simulink model "model_knigge"  (R2020b)
settings: configuration reference "Configuration" (kept outside this file)
settings Model: Creator=dogukan  LastModifiedBy=dogukan
settings ConfigSetRef: SourceName=Configuration  SourceLocation=Base Workspace

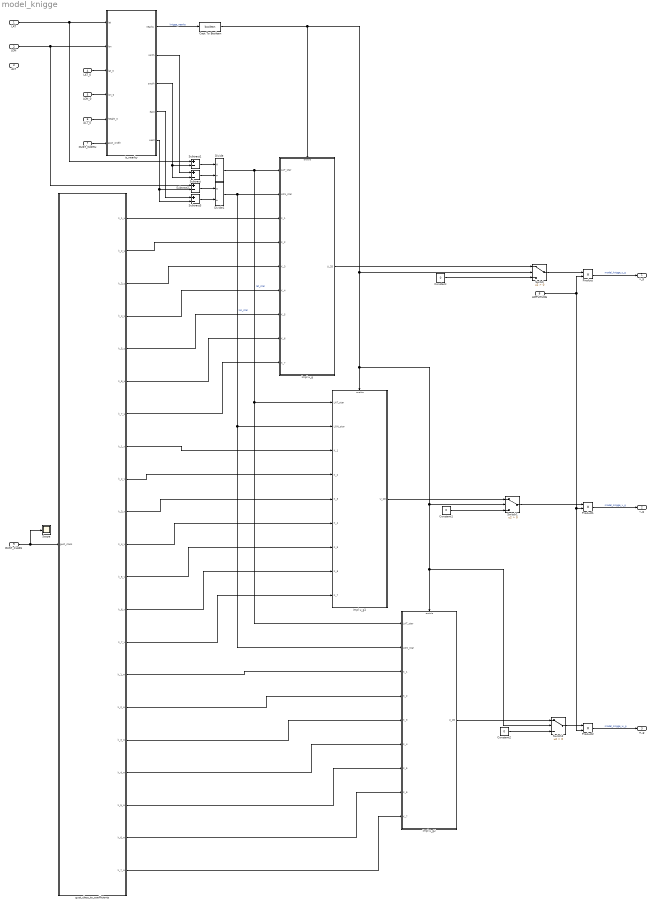
== system model_knigge ==
  LAT : Inport
  LON : Inport  Port=2
  ALT : Inport  Port=3
  LAT_0 : Inport  Port=4
  LON_0 : Inport  Port=5
  ALT_0 : Inport  Port=6
  GUST_WIDTH : Inport  Port=7
  AMPLITUDE : Inport  Port=8
  GUST_CLASS : Inport  Port=9
  Cast To Boolean : DataTypeConversion  OutDataTypeStr=boolean
  Constant : Constant  Value=0
  Constant1 : Constant  Value=0
  Constant2 : Constant  Value=0
  Divide : Product  Inputs=*/
  Divide1 : Product  Inputs=*/
  Product : Product
  Product1 : Product
  Product2 : Product
  Scope : Scope
  Subtract{,1..3} (4 alike) : Sum  Inputs=+-
  Switch : Switch  Criteria=u2 > Threshold
  Switch1 : Switch  Criteria=u2 > Threshold
  Switch2 : Switch  Criteria=u2 > Threshold
  gust_class_to_coefficients : MATLAB Function  TreatAsAtomicUnit=on
  impl u_g : Subsystem  TreatAsAtomicUnit=on
  impl u_g1 : Subsystem  TreatAsAtomicUnit=on
  impl u_g2 : Subsystem  TreatAsAtomicUnit=on
  is_nearby : MATLAB Function  TreatAsAtomicUnit=on
  u_g : Outport
  v_g : Outport  Port=2
  w_g : Outport  Port=3
  wires:
  LAT/1 -> is_nearby/1(lat), Subtract1/1
  LON/1 -> is_nearby/2(lon), Subtract2/1
  is_nearby/1(nearby) -> Cast To Boolean/1  "knigge_nearby"
  impl u_g/1(U_2D) -> Switch/1
  Cast To Boolean/1 -> impl u_g/Enable, impl u_g2/Enable, Switch2/2, Switch1/2, impl u_g1/Enable, Switch/2
  Constant/1 -> Switch/3
  LAT_0/1 -> is_nearby/3(lat_0)
  LON_0/1 -> is_nearby/4(lon_0)
  ALT_0/1 -> is_nearby/5(height_0)
  GUST_WIDTH/1 -> is_nearby/6(gust_width)
  Divide/1 -> impl u_g2/1(LAT_star), impl u_g1/1(LAT_star), impl u_g/1(LAT_star)  "lat_star"
  is_nearby/2(north) -> Subtract/1
  is_nearby/3(south) -> Subtract/2, Subtract1/2
  Subtract/1 -> Divide/2
  Subtract1/1 -> Divide/1
  Divide1/1 -> impl u_g2/2(LON_star), impl u_g1/2(LON_star), impl u_g/2(LON_star)  "lon_star"
  Subtract2/1 -> Divide1/1
  Subtract3/1 -> Divide1/2
  is_nearby/4(east) -> Subtract3/1
  is_nearby/5(west) -> Subtract3/2, Subtract2/2
  gust_class_to_coefficients/2(k_2_u) -> impl u_g/4(K_2)
  gust_class_to_coefficients/1(k_1_u) -> impl u_g/3(K_1)
  gust_class_to_coefficients/3(k_3_u) -> impl u_g/5(K_3)
  gust_class_to_coefficients/4(k_4_u) -> impl u_g/6(K_4)
  gust_class_to_coefficients/5(k_5_u) -> impl u_g/7(K_5)
  gust_class_to_coefficients/6(k_6_u) -> impl u_g/8(K_6)
  gust_class_to_coefficients/7(k_7_u) -> impl u_g/9(K_7)
  GUST_CLASS/1 -> Scope/1, gust_class_to_coefficients/1(gust_class)
  gust_class_to_coefficients/8(k_1_v) -> impl u_g1/3(K_1)
  gust_class_to_coefficients/9(k_2_v) -> impl u_g1/4(K_2)
  gust_class_to_coefficients/10(k_3_v) -> impl u_g1/5(K_3)
  gust_class_to_coefficients/11(k_4_v) -> impl u_g1/6(K_4)
  gust_class_to_coefficients/12(k_5_v) -> impl u_g1/7(K_5)
  gust_class_to_coefficients/13(k_6_v) -> impl u_g1/8(K_6)
  gust_class_to_coefficients/14(k_7_v) -> impl u_g1/9(K_7)
  impl u_g1/1(U_2D) -> Switch1/1
  Constant1/1 -> Switch1/3
  Switch1/1 -> Product1/1
  gust_class_to_coefficients/15(k_1_w) -> impl u_g2/3(K_1)
  gust_class_to_coefficients/16(k_2_w) -> impl u_g2/4(K_2)
  gust_class_to_coefficients/17(k_3_w) -> impl u_g2/5(K_3)
  gust_class_to_coefficients/18(k_4_w) -> impl u_g2/6(K_4)
  gust_class_to_coefficients/19(k_5_w) -> impl u_g2/7(K_5)
  gust_class_to_coefficients/20(k_6_w) -> impl u_g2/8(K_6)
  gust_class_to_coefficients/21(k_7_w) -> impl u_g2/9(K_7)
  impl u_g2/1(U_2D) -> Switch2/1
  Constant2/1 -> Switch2/3
  Switch2/1 -> Product2/1
  Switch/1 -> Product/1
  Product/1 -> u_g/1  "model_knigge_u_g"
  AMPLITUDE/1 -> Product2/2, Product1/2, Product/2
  Product1/1 -> v_g/1  "model_knigge_v_g"
  Product2/1 -> w_g/1  "model_knigge_w_g"

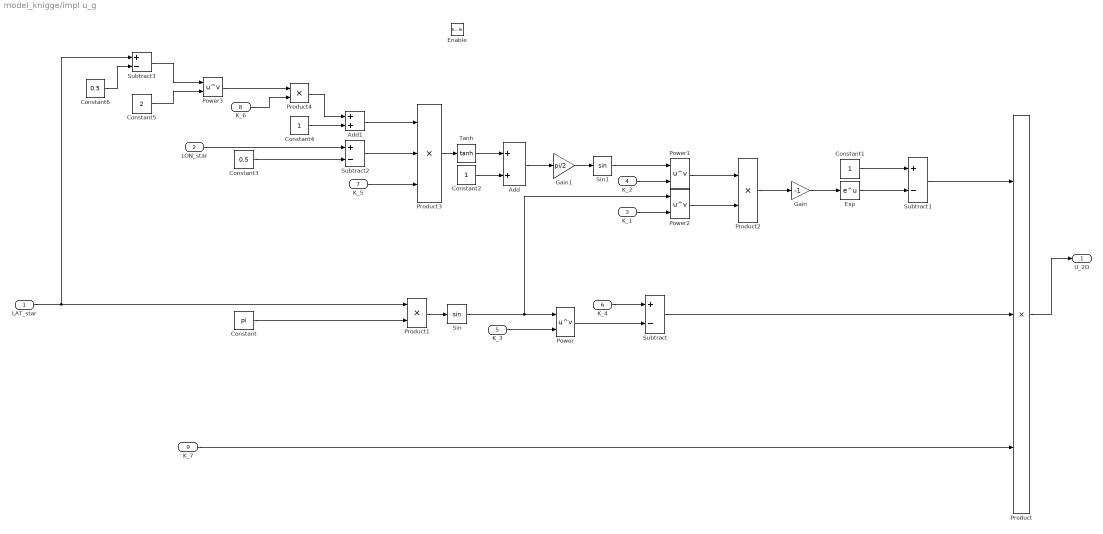
== system model_knigge/impl u_g ==
  LAT_star : Inport
  LON_star : Inport  Port=2
  K_1 : Inport  Port=3
  K_2 : Inport  Port=4
  K_3 : Inport  Port=5
  K_4 : Inport  Port=6
  K_5 : Inport  Port=7
  K_6 : Inport  Port=8
  K_7 : Inport  Port=9
  Enable : EnablePort
  Add : Sum
  Add1 : Sum
  Constant : Constant  Value=pi
  Constant1 : Constant
  Constant2 : Constant
  Constant3 : Constant  Value=0.5
  Constant4 : Constant
  Constant5 : Constant  Value=2
  Constant6 : Constant  Value=0.5
  Exp : Math  SaturateOnIntegerOverflow=on
  Gain : Gain  Gain=-1
  Gain1 : Gain  Gain=pi/2
  Power{,1..3} (4 alike) : Math  Operator=pow  SaturateOnIntegerOverflow=on
  Product : Product  Inputs=3
  Product1 : Product
  Product2 : Product
  Product3 : Product  Inputs=3
  Product4 : Product
  Sin : Trigonometry
  Sin1 : Trigonometry
  Subtract{,1..3} (4 alike) : Sum  Inputs=+-
  Tanh : Trigonometry  Operator=tanh
  U_2D : Outport
  wires:
  K_7/1 -> Product/3
  K_3/1 -> Power/2
  K_4/1 -> Subtract/1
  Power/1 -> Subtract/2
  Subtract/1 -> Product/2
  LAT_star/1 -> Subtract3/1, Product1/1
  Constant/1 -> Product1/2
  Product1/1 -> Sin/1
  Constant1/1 -> Subtract1/1
  Subtract1/1 -> Product/1
  Exp/1 -> Subtract1/2
  Gain/1 -> Exp/1
  Product2/1 -> Gain/1
  Power1/1 -> Product2/1
  Power2/1 -> Product2/2
  K_2/1 -> Power1/2
  K_1/1 -> Power2/2
  Sin1/1 -> Power1/1
  Sin/1 -> Power2/1, Power/1
  Gain1/1 -> Sin1/1
  Add/1 -> Gain1/1
  Constant2/1 -> Add/2
  Tanh/1 -> Add/1
  Product3/1 -> Tanh/1
  K_5/1 -> Product3/3
  Subtract2/1 -> Product3/2
  LON_star/1 -> Subtract2/1
  Constant3/1 -> Subtract2/2
  Add1/1 -> Product3/1
  Constant4/1 -> Add1/2
  Product4/1 -> Add1/1
  K_6/1 -> Product4/2
  Constant5/1 -> Power3/2
  Power3/1 -> Product4/1
  Constant6/1 -> Subtract3/2
  Subtract3/1 -> Power3/1
  Product/1 -> U_2D/1

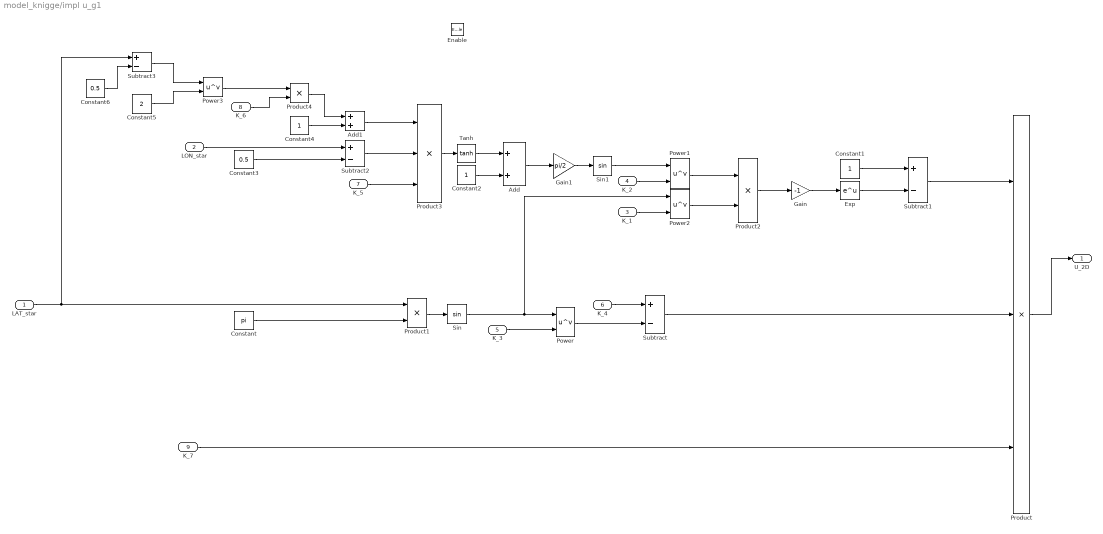
== system model_knigge/impl u_g1 ==
  LAT_star : Inport
  LON_star : Inport  Port=2
  K_1 : Inport  Port=3
  K_2 : Inport  Port=4
  K_3 : Inport  Port=5
  K_4 : Inport  Port=6
  K_5 : Inport  Port=7
  K_6 : Inport  Port=8
  K_7 : Inport  Port=9
  Enable : EnablePort
  Add : Sum
  Add1 : Sum
  Constant : Constant  Value=pi
  Constant1 : Constant
  Constant2 : Constant
  Constant3 : Constant  Value=0.5
  Constant4 : Constant
  Constant5 : Constant  Value=2
  Constant6 : Constant  Value=0.5
  Exp : Math  SaturateOnIntegerOverflow=on
  Gain : Gain  Gain=-1
  Gain1 : Gain  Gain=pi/2
  Power{,1..3} (4 alike) : Math  Operator=pow  SaturateOnIntegerOverflow=on
  Product : Product  Inputs=3
  Product1 : Product
  Product2 : Product
  Product3 : Product  Inputs=3
  Product4 : Product
  Sin : Trigonometry
  Sin1 : Trigonometry
  Subtract{,1..3} (4 alike) : Sum  Inputs=+-
  Tanh : Trigonometry  Operator=tanh
  U_2D : Outport
  wires:
  K_7/1 -> Product/3
  K_3/1 -> Power/2
  K_4/1 -> Subtract/1
  Power/1 -> Subtract/2
  Subtract/1 -> Product/2
  LAT_star/1 -> Subtract3/1, Product1/1
  Constant/1 -> Product1/2
  Product1/1 -> Sin/1
  Constant1/1 -> Subtract1/1
  Subtract1/1 -> Product/1
  Exp/1 -> Subtract1/2
  Gain/1 -> Exp/1
  Product2/1 -> Gain/1
  Power1/1 -> Product2/1
  Power2/1 -> Product2/2
  K_2/1 -> Power1/2
  K_1/1 -> Power2/2
  Sin1/1 -> Power1/1
  Sin/1 -> Power2/1, Power/1
  Gain1/1 -> Sin1/1
  Add/1 -> Gain1/1
  Constant2/1 -> Add/2
  Tanh/1 -> Add/1
  Product3/1 -> Tanh/1
  K_5/1 -> Product3/3
  Subtract2/1 -> Product3/2
  LON_star/1 -> Subtract2/1
  Constant3/1 -> Subtract2/2
  Add1/1 -> Product3/1
  Constant4/1 -> Add1/2
  Product4/1 -> Add1/1
  K_6/1 -> Product4/2
  Constant5/1 -> Power3/2
  Power3/1 -> Product4/1
  Constant6/1 -> Subtract3/2
  Subtract3/1 -> Power3/1
  Product/1 -> U_2D/1

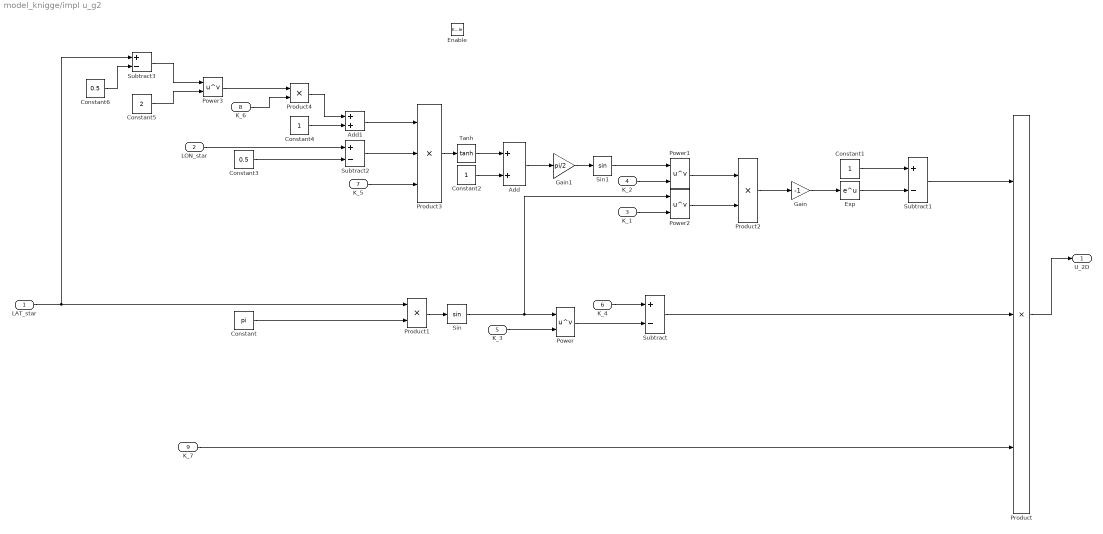
== system model_knigge/impl u_g2 ==
  LAT_star : Inport
  LON_star : Inport  Port=2
  K_1 : Inport  Port=3
  K_2 : Inport  Port=4
  K_3 : Inport  Port=5
  K_4 : Inport  Port=6
  K_5 : Inport  Port=7
  K_6 : Inport  Port=8
  K_7 : Inport  Port=9
  Enable : EnablePort
  Add : Sum
  Add1 : Sum
  Constant : Constant  Value=pi
  Constant1 : Constant
  Constant2 : Constant
  Constant3 : Constant  Value=0.5
  Constant4 : Constant
  Constant5 : Constant  Value=2
  Constant6 : Constant  Value=0.5
  Exp : Math  SaturateOnIntegerOverflow=on
  Gain : Gain  Gain=-1
  Gain1 : Gain  Gain=pi/2
  Power{,1..3} (4 alike) : Math  Operator=pow  SaturateOnIntegerOverflow=on
  Product : Product  Inputs=3
  Product1 : Product
  Product2 : Product
  Product3 : Product  Inputs=3
  Product4 : Product
  Sin : Trigonometry
  Sin1 : Trigonometry
  Subtract{,1..3} (4 alike) : Sum  Inputs=+-
  Tanh : Trigonometry  Operator=tanh
  U_2D : Outport
  wires:
  K_7/1 -> Product/3
  K_3/1 -> Power/2
  K_4/1 -> Subtract/1
  Power/1 -> Subtract/2
  Subtract/1 -> Product/2
  LAT_star/1 -> Subtract3/1, Product1/1
  Constant/1 -> Product1/2
  Product1/1 -> Sin/1
  Constant1/1 -> Subtract1/1
  Subtract1/1 -> Product/1
  Exp/1 -> Subtract1/2
  Gain/1 -> Exp/1
  Product2/1 -> Gain/1
  Power1/1 -> Product2/1
  Power2/1 -> Product2/2
  K_2/1 -> Power1/2
  K_1/1 -> Power2/2
  Sin1/1 -> Power1/1
  Sin/1 -> Power2/1, Power/1
  Gain1/1 -> Sin1/1
  Add/1 -> Gain1/1
  Constant2/1 -> Add/2
  Tanh/1 -> Add/1
  Product3/1 -> Tanh/1
  K_5/1 -> Product3/3
  Subtract2/1 -> Product3/2
  LON_star/1 -> Subtract2/1
  Constant3/1 -> Subtract2/2
  Add1/1 -> Product3/1
  Constant4/1 -> Add1/2
  Product4/1 -> Add1/1
  K_6/1 -> Product4/2
  Constant5/1 -> Power3/2
  Power3/1 -> Product4/1
  Constant6/1 -> Subtract3/2
  Subtract3/1 -> Power3/1
  Product/1 -> U_2D/1

== matlab function model_knigge/is_nearby ==
  data: lat input; nearby output; lon input; lat_0 input; lon_0 input; height_0 input; gust_width input; north output; south output; east output; west output
% model_knigge
function [nearby, north, south, east, west] = is_nearby(lat, lon, lat_0, lon_0, height_0, gust_width)
    % Units:
    % [lat] = rad
    % [lon] = rad
    % [lat_0] = rad
    % [lon_0] = rad
    % [height_0] = m
    % [gust_width] = m
    % Independet of altitude, phenomena is available on all heights, because otherwise height distribution is needed

    % Option 1: doesn't support code gen
    % [arclen, az] = distance(lat, lon, lat0, lon0);
    % nearby = arclen < width;

    % Option 2: ¯\_(ツ)_/¯
    % earth_radius = 6371000; % m
    % delta_phi = lat - lat_0;
    % delta_lambda = lon - lon_0;
    % a = sin(delta_phi / 2) ^ 2 + cos(lat) * cos(lat_0) * cos(delta_lambda / 2) ^ 2;
    % c = 2 * atan2(sqrt(a), sqrt(1 - a));
    % dist = earth_radius * c;
    % nearby = dist < width;

    % Option 3:
    north_lla = ned2lla([gust_width/2, 0, 0], [lat_0, lon_0, height_0], "flat");
    north = deg2rad(north_lla(1)); % rad
    south_lla = ned2lla([-gust_width/2, 0, 0], [lat_0, lon_0, height_0], "flat");
    south = deg2rad(south_lla(1)); % rad
    inside_lat = (south < lat) & (lat < north);
    % disp(inside_lat);

    east_lla = ned2lla([0, gust_width/2, 0], [lat_0, lon_0, height_0], "flat");
    east = deg2rad(east_lla(2)); % rad
    west_lla = ned2lla([0, -gust_width/2, 0], [lat_0, lon_0, height_0], "flat");
    west = deg2rad(west_lla(2)); % rad
    inside_lon = (west < lon) & (lon < east);
    % disp(inside_lon);

    nearby = inside_lat & inside_lon;
end

== matlab function model_knigge/gust_class_to_coefficients ==
  data: gust_class input; k_1_u output; k_2_u output; k_3_u output; k_4_u output; k_5_u output; k_6_u output; k_7_u output; k_1_v output; k_2_v output; k_3_v output; k_4_v output; k_5_v output; k_6_v output; k_7_v output; k_1_w output; k_2_w output; k_3_w output; k_4_w output; k_5_w output; k_6_w output; k_7_w output
function [k_1_u, k_2_u, k_3_u, k_4_u, k_5_u, k_6_u, k_7_u, ...
    k_1_v, k_2_v, k_3_v, k_4_v, k_5_v, k_6_v, k_7_v, ...
    k_1_w, k_2_w, k_3_w, k_4_w, k_5_w, k_6_w, k_7_w] = gust_class_to_coefficients(gust_class)
%     gust_class = gust_class_vector(2);
%     disp(gust_class_vector);
    if gust_class == 1
        k_1_u = 1.9;
        k_2_u = 4.6;
        k_3_u = 0.12;
        k_4_u = 1.08;
        k_5_u = 2.3;
        k_6_u = 2.0;
        k_7_u = 19.2;
        k_1_v = 1.9;
        k_2_v = 4.6;
        k_3_v = 0.12;
        k_4_v = 1.08;
        k_5_v = 2.3;
        k_6_v = 2.0;
        k_7_v = 19.2;
        k_1_w = 1.5;
        k_2_w = 1.3;
        k_3_w = 3.0;
        k_4_w = 5.0;
        k_5_w = 5.0;
        k_6_w = 1.0;
        k_7_w = 0.395;
    elseif gust_class == 2
        k_1_u = 1.2;
        k_2_u = 1.4;
        k_3_u = 0.2;
        k_4_u = 1.2;
        k_5_u = 5.4;
        k_6_u = 1.5;
        k_7_u = 7.7;
        k_1_v = 1.2;
        k_2_v = 1.4;
        k_3_v = 0.2;
        k_4_v = 1.2;
        k_5_v = 5.4;
        k_6_v = 1.5;
        k_7_v = 7.7;
        k_1_w = 1.5;
        k_2_w = 1.4;
        k_3_w = 0.2;
        k_4_w = 1.18;
        k_5_w = 5.1;
        k_6_w = 1.1;
        k_7_w = 8.5;        
    else  % gust_class == 3
        k_1_u = 1.2;
        k_2_u = 1.4;
        k_3_u = 0.2;
        k_4_u = 1.2;
        k_5_u = 5.4;
        k_6_u = 1.5;
        k_7_u = 7.7;
        k_1_v = 1.2;
        k_2_v = 1.4;
        k_3_v = 0.2;
        k_4_v = 1.2;
        k_5_v = 5.4;
        k_6_v = 1.5;
        k_7_v = 7.7;
        k_1_w = 1.3;
        k_2_w = 1.1;
        k_3_w = 0.1;
        k_4_w = 1.07;
        k_5_w = 6.0;
        k_6_w = 1.2;
        k_7_w = 19.0;
    end
end
